simulink model "Regen1"  (Simulink 6.5)
settings: Solver=FixedStepDiscrete  StartTime=0.0  StopTime=1  FixedStep=Ts  RelTol=1e-3  AbsTol=1e-3
PreLoadFcn:
  | assignin('base','Ts',[2e-6])
undefined symbols (not defined in the file): DiscIntNeverNeededParam, powergui, Ts, x
libraries: powerlib x18, powerlib_extras x8
settings Model: Creator=sybille  LastModifiedBy=RS  ExtModeTrigMode=oneshot  ExtModeArmWhenConnect=off  ExtModeAutoUpdateStatusClock=off
settings DataIOCC: LimitDataPoints=off  SaveOutput=off  SaveTime=off  SignalLoggingName=sigsOut
settings OptimizationCC: BlockReduction=off  BooleanDataType=off  InlineInvariantSignals=on
settings DebuggingCC: CheckExecutionContextPreStartOutputMsg=on  CheckExecutionContextRuntimeOutputMsg=on  SolverPrmCheckMsg=none  MultiTaskDSMMsg=warning  MultiTaskCondExecSysMsg=none  StrictBusMsg=None
settings HardwareCC: TargetUnknown=on
settings RTWCC: IncludeERTFirstTime=on

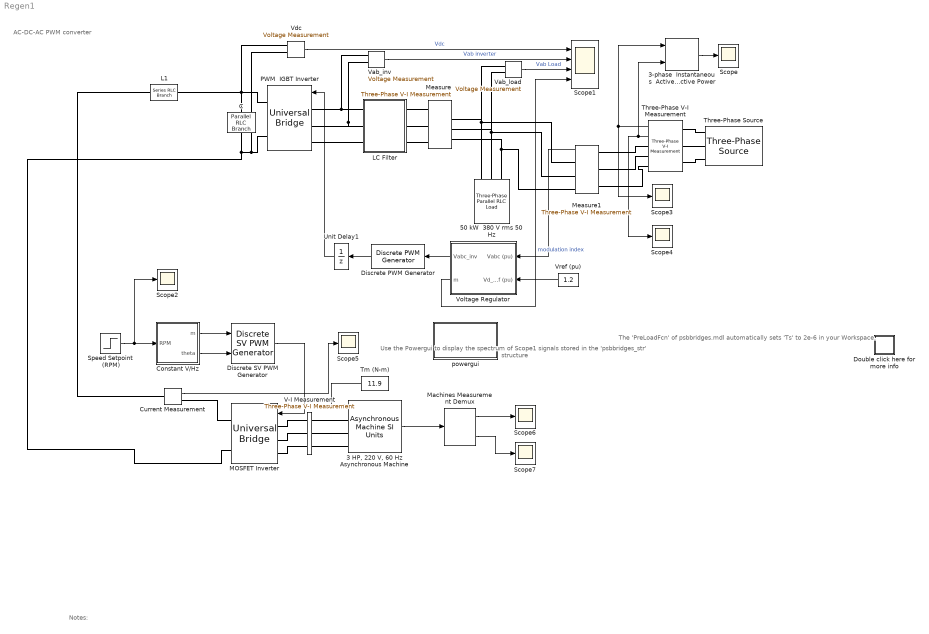
== system Regen1 ==
  note: AC-DC-AC PWM converter
  note: The 'PreLoadFcn' of psbbridges.mdl
      | automatically sets 'Ts' to 2e-6 in your Workspace.
  note: Use the Powergui to display
      | the spectrum of Scope1 signals
      | stored in the  'psbbridges_str'
      | structure
  note: Notes:
  "3 HP, 220 V, 60 Hz Asynchronous Machine" : powerlib/Machines/Asynchronous Machine SI Units  DialogController=PMDialogs.PMDefaultMaskDlg  SystemSampleTime=-1  PresetModel=No  MechanicalLoad=Torque Tm  ShowDetailedParameters=on  RotorType=Squirrel-cage  ReferenceFrame=Stationary  NominalParameters=[ 3*746, 220, 60 ]  Stator="[ 0.435  2*2.0e-3 ]"  Rotor="[ 0.816  2.0e-3 ]"  Lm=69.31e-3  Mechanical="[ 0.089  0  2 ]"  PolePairs=2  InitialConditions=[0.044533 0 11.138 11.138 11.138 -39.6 -159.6 80.4]  Units=1  LoadFlowParameters=2000  SimulateSaturation=off  Saturation=[0 0;0 0]
  3-phase  Instantaneous  Active & Reactive Power : powerlib_extras/Measurements/3-phase  Instantaneous  Active & Reactive Power  DialogController=PMDialogs.PMDefaultMaskDlg  SystemSampleTime=-1
  50 kW  380 V rms 50 Hz : powerlib/Elements/Three-Phase Parallel RLC Load  Orientation=down  DialogController=PMDialogs.PMDefaultMaskDlg  PhysicalDomain=powersysdomain  SubClassName=unknown  LeftPortType=p1  RightPortType=p1  LConnTagsString=A|B|C  Configuration=Y (grounded)  NominalVoltage=380  NominalFrequency=50  ActivePower=0  InductivePower=0  CapacitivePower=0  Measurements=None
  C : powerlib/Elements/Parallel RLC Branch  Orientation=down  DialogController=PMDialogs.PMDefaultMaskDlg  PhysicalDomain=powersysdomain  SubClassName=unknown  LeftPortType=p1  RightPortType=p1  LConnTagsString=a  RConnTagsString=__new0  BranchType=C  Resistance=1.0  Inductance=1.0  SetiL0=off  InitialCurrent=0  Capacitance=5000e-06  Setx0=off  InitialVoltage=0  Measurements=None
  Constant V/Hz : Subsystem
  Current Measurement : powerlib/Measurements/Current Measurement  DialogController=PMDialogs.PMDefaultMaskDlg  SystemSampleTime=-1  PhasorSimulation=off  OutputType=Complex  PSBequivalent=0
  Discrete PWM Generator : powerlib_extras/Discrete  Control Blocks/Discrete PWM Generator  Orientation=left  DialogController=PMDialogs.PMDefaultMaskDlg  SystemSampleTime=-1  GeneratorMode="3-arm  bridge (6 pulses)"  Fc=2000  Ts=Ts  Internal=off  mIndex=0.4  Freq=60  Phase=0
  Discrete SV PWM Generator : powerlib_extras/Discrete  Control Blocks/Discrete SV PWM Generator  DialogController=PMDialogs.PMDefaultMaskDlg  SystemSampleTime=-1  InputType=Magnitude-Angle (rad)  SwitchingPattern=Pattern #1  Fc=1980  ParUref=[0.8 -30 50]  Ts=Ts
  Double click here for more info : Subsystem
      settings: OpenFcn=showdemo(bdroot(gcb))
      mask Display: disp('?')
  L1 : powerlib/Elements/Series RLC Branch  DialogController=PMDialogs.PMDefaultMaskDlg  PhysicalDomain=powersysdomain  SubClassName=unknown  LeftPortType=p1  RightPortType=p1  LConnTagsString=__new0  RConnTagsString=__new0  BranchType=L  Resistance=1.0  Inductance=200e-6  SetiL0=off  InitialCurrent=0  Capacitance=1.0  Setx0=off  InitialVoltage=0  Measurements=None
  LC Filter : Subsystem
  MOSFET Inverter : powerlib/Power Electronics/Universal Bridge  Orientation=left  DialogController=PMDialogs.PMDefaultMaskDlg  SystemSampleTime=-1  Arms=3  SnubberResistance=1e5  SnubberCapacitance=inf  Device=MOSFET / Diodes  Ron=0.2e-3  Lon=0  ForwardVoltages="[  0  0  ]"  ForwardVoltage=0  GTOparameters=[ 10e-6 , 20e-6 ]  IGBTparameters=[ 1e-6 , 2e-6 ]  Measurements=None  converterType=Rectifier
  Machines Measurement Demux : powerlib/Machines/Machines Measurement Demux  DialogController=PMDialogs.PMDefaultMaskDlg  SystemSampleTime=-1  machType=Asynchronous  ssm1=on  ssm2=on  ssm3=on  ssm4=on  ssm5=on  ssm6=on  sm1=off  sm2=off  sm3=off  sm4=off  sm5=off  sm6=off  sm7=off  sm8=on  sm9=off  sm10=off  sm11=off  sm115=off  sm12=off  sm13=off  sm14=off  asm1=off  asm2=off  asm3=off  asm4=off  asm5=on  asm6=off  asm7=off  asm8=off  asm9=on  asm10=off  asm11=off  pmsm1=on  pmsm2=on  pmsm3=on  pmsm4=off  pmsm5=on  pmsm6=on  pmsm7=on  lastType=1
  Measure : powerlib/Measurements/Three-Phase V-I Measurement  DialogController=PMDialogs.PMDefaultMaskDlg  SystemSampleTime=-1  VoltageMeasurement=phase-to-ground  SetLabelV=off  LabelV=V1  Vpu=on  CurrentMeasurement=no  SetLabelI=off  LabelI=I1  Ipu=off  Pbase=1e3  Vbase=380  OutputType=Magnitude  PhasorSimulation=off  PSBequivalent=0
  Measure1 : powerlib/Measurements/Three-Phase V-I Measurement  Orientation=left  DialogController=PMDialogs.PMDefaultMaskDlg  SystemSampleTime=-1  VoltageMeasurement=phase-to-ground  SetLabelV=off  LabelV=V1  Vpu=on  CurrentMeasurement=no  SetLabelI=off  LabelI=I1  Ipu=off  Pbase=1e3  Vbase=380  OutputType=Magnitude  PhasorSimulation=off  PSBequivalent=0
  PWM  IGBT Inverter : powerlib/Power Electronics/Universal Bridge  Orientation=left  DialogController=PMDialogs.PMDefaultMaskDlg  SystemSampleTime=-1  Arms=3  SnubberResistance=5000  SnubberCapacitance=inf  Device=IGBT / Diodes  Ron=1e-3  Lon=0  ForwardVoltages="[  0.0  0.0  ]"  ForwardVoltage=.8  GTOparameters=[ 1e-6 ,1e-6 ]  IGBTparameters=[ 1e-6 , 2e-6 ]  Measurements=Device currents  converterType=Rectifier
  Scope{,2..7} (7 alike) : Scope
      Scope settings: MaxDataPoints=10000000  SampleInput=on  SampleTime=2e-6
      Scope2 settings: MaxDataPoints=10000000  SampleInput=on  SampleTime=2e-6
      Scope3 settings: SaveName=ScopeData2  MaxDataPoints=10000000  SampleInput=on  SampleTime=2e-6
      Scope4 settings: SaveName=ScopeData3  MaxDataPoints=10000000  SampleInput=on  SampleTime=2e-6
      Scope5 settings: SaveName=ScopeData4  MaxDataPoints=10000000  SampleInput=on  SampleTime=2e-6
      Scope6 settings: SaveName=ScopeData5  MaxDataPoints=10000000  SampleInput=on  SampleTime=2e-6
      Scope7 settings: YMin=124.5  YMax=127.25  SaveName=ScopeData6  MaxDataPoints=10000000  SampleInput=on  SampleTime=2e-6
  Scope1 : Scope  NumInputPorts=4
      settings: TimeRange=0.1  YMin=0~-1500~-750~0.4  YMax=1100~1500~750~1.1  SaveName=psbbridges_str
  Speed Setpoint (RPM) : Step  Time=0.5  After=1300  SampleTime=Ts
  Three-Phase V-I Measurement : powerlib/Measurements/Three-Phase V-I Measurement  Orientation=left  DialogController=PMDialogs.PMDefaultMaskDlg  SystemSampleTime=-1  VoltageMeasurement=phase-to-ground  SetLabelV=off  LabelV=Vabc  Vpu=off  CurrentMeasurement=yes  SetLabelI=off  LabelI=Iabc  Ipu=off  Pbase=100e6  Vbase=500e3  OutputType=Complex  PhasorSimulation=off  PSBequivalent=0
  Three-Phase Source : powerlib/Electrical Sources/Three-Phase Source  Orientation=left  DialogController=PMDialogs.PMDefaultMaskDlg  SystemSampleTime=-1  Voltage=390  PhaseAngle=0  Frequency=50  InternalConnection=Yg  SpecifyImpedance=off  Resistance=0.00001  Inductance=0.00001  ShortCircuitLevel=100e6  BaseVoltage=25e3  XRratio=7
  Tm (N-m) : Constant  Orientation=left  Value=11.9  OutDataType=sfix(16)  ConRadixGroup=Use specified scaling  OutScaling=2^0  SampleTime=inf  FramePeriod=inf
  Unit Delay1 : UnitDelay  Orientation=left  SampleTime=Ts
  V-I Measurement : powerlib/Measurements/Three-Phase V-I Measurement  DialogController=PMDialogs.PMDefaultMaskDlg  SystemSampleTime=-1  VoltageMeasurement=phase-to-phase  SetLabelV=on  LabelV=Vabc_Stator  Vpu=off  CurrentMeasurement=yes  SetLabelI=on  LabelI=Iabc_Stator  Ipu=off  Pbase=100e6  Vbase=500e3  OutputType=Magnitude  PhasorSimulation=off  PSBequivalent=0
  Vab_inv : powerlib/Measurements/Voltage Measurement  Tag=PoWeRsYsTeMmEaSuReMeNt  DialogController=PMDialogs.PMDefaultMaskDlg  SystemSampleTime=-1  PhasorSimulation=off  OutputType=Magnitude  PSBequivalent=0
  Vab_load : powerlib/Measurements/Voltage Measurement  Tag=PoWeRsYsTeMmEaSuReMeNt  DialogController=PMDialogs.PMDefaultMaskDlg  SystemSampleTime=-1  PhasorSimulation=off  OutputType=Magnitude  PSBequivalent=0
  Vdc : powerlib/Measurements/Voltage Measurement  Tag=PoWeRsYsTeMmEaSuReMeNt  DialogController=PMDialogs.PMDefaultMaskDlg  SystemSampleTime=-1  PhasorSimulation=off  OutputType=Magnitude  PSBequivalent=0
  Voltage Regulator : Subsystem  Orientation=left  mask( Voltage Regulator){Kp=0.4, Ki=500, Ts=Ts}
      mask prompts: Kp "Proportional gain  Kp:"; Ki "Integral gain Ki:"; Ts "Sample time (s) :"
  "Vref (pu) " : Constant  Orientation=left  Value=1.2  OutDataType=sfix(16)  ConRadixGroup=Use specified scaling  OutScaling=2^0  SampleTime=inf  FramePeriod=inf
  powergui : Subsystem  Priority=2  AncestorBlock=powerlib/powergui  InitFcn=powergui( 'InitFcn_Callback' , gcb , 0 , [ ] );  mask(PSB option menu block){SimulationMode=Discrete, SampleTime=Ts, echomessages=on, RestoreLinks=warning, x0status=blocks, Frange=[0:2:500], Ylog=off, Xlog=on, ShowGrid=off, save=off, variable=ZData, structure=psbbridges_str, ZoomFFT=on, StartTime=0.1-2/50, cycles=2, DisplayStyle=off, fundamental=50, FreqAxis=off, MaxFrequency=7000, frequencyindice=60, frequencyindicesteady=1, RmsSteady=1, display=off, Ts=0, frequency=60, methode=off, HookPort=off, Interpol=off}
      mask prompts: SimulationMode "Simulation mode"; SampleTime "Sample time Ts (when simulation mode is Discrete) (s)"; echomessages "Echo  Messages"; RestoreLinks "Restore disabled links"; x0status "Initial electrical states status"; Frange "Impedance tool: Frequency Range"; Ylog "Impedance tool: Log impedance"; Xlog "Impedance tool: log Frequency"; ShowGrid "Impedance tool: grid"; save "Impedance tool: Save Data To Workspace"; variable "Impedance tool: Variable Name"; structure "Structure Name (PSBFFTSCOPE)"; ZoomFFT "ZoomFFT (PSBFFTSCOPE)"; StartTime "Start Time (PSBFFTSCOPE)"; cycles "Cycles (PSBFFTSCOPE)"; DisplayStyle "Display style (PSBFFTSCOPE)"; fundamental "Fundamental (PSBFFTSCOPE)"; FreqAxis "Frequency Axis (PSBFFTSCOPE)"; MaxFrequency "Max Frequency (PSBFFTSCOPE)"; frequencyindice "Load flow frequency (Hz)"; frequencyindicesteady "Frequency indice (STEADYSTATE)"; RmsSteady "RMS display (STEADYSTATE)"; display "Display Results"; Ts "OBSOLETE 1"; frequency "Phasor frequency (Hz)"; methode "Phasor simulation"; HookPort "Hook port"; Interpol "Interpolate"
      mask init:
      | powerlibroot = which('powersysdomain');
      | PSBroot = powerlibroot(1:end-16);
      | %
      | switch SimulationMode
      | 	case 1
      | 		message=sprintf('Continuous');
      | 	case 2
      |         SampleTimeeval=evalin('base',SampleTime,'NaN');
      |         if isnan(SampleTimeeval)
      |             message=sprintf('Warning !!,\nUndefined sample time');
      |         else
      |             message=sprintf('Discrete,\nTs = %.4g s.',SampleTimeeval);
      |         end
      | 	case 3
      | 		message=sprintf('Phasors');
      | end
      | if strcmp(bdroot,'powerlib')
      |   message='powergui';
      | end
      | power_initmask();
      settings: CopyFcn=powergui( 'Copy_Callback' , gcb , 0 , [ ] );  ModelCloseFcn=powergui( 'CloseButton_Callback' , gcb , [ ] , [ ] );  PreSaveFcn=powergui( 'CloseButton_Callback' , gcb , [ ] , [ ] );  NameChangeFcn=powergui( 'NameChangeFcn_Callback' , gcb , 0 , [ ] );
      settings: DeleteFcn=|
      | powergui( 'Copy_Callback' , gcb , 1 , [ ] );
      | powergui( 'CloseButton_Callback' , gcb , [ ] , [ ] );
      settings: OpenFcn=|
      | if (power_openblockproxy ('secondary'))
      | powergui(gcb,'PM')
      | end;
      mask Help: web(psbhelp)
      mask StyleString: popup(Continuous|Discrete|Phasor),edit,checkbox,popup(yes|warning|no),popup(blocks|steady|zero),edit,checkbox,checkbox,checkbox,checkbox,edit,edit,checkbox,edit,edit,edit,edit,checkbox,edit,edit,edit,edit,checkbox,edit,edit,checkbox,checkbox,checkbox
      mask CallbackString: ||||||||||||||||||||||||||powergui('HookPort',[],[],gcb);|
      mask Display: disp(message)
  wires:
  "Vref (pu) "/1 -> Voltage Regulator/2(Vd_ref (pu))
  Discrete PWM Generator/1 -> Unit Delay1/1
  Voltage Regulator/1(Vabc_inv) -> Discrete PWM Generator/1
  Voltage Regulator/2(m) -> Scope1/4  "modulation index"
  Vdc/1 -> Scope1/1  "Vdc"
  Vab_load/1 -> Scope1/3  "Vab Load"
  Vab_inv/1 -> Scope1/2  "Vab inverter"
  Unit Delay1/1 -> PWM  IGBT Inverter/1
  3-phase  Instantaneous  Active & Reactive Power/1 -> Scope/1
  Three-Phase V-I Measurement/1 -> Scope3/1, 3-phase  Instantaneous  Active & Reactive Power/1
  Three-Phase V-I Measurement/2 -> Scope4/1, 3-phase  Instantaneous  Active & Reactive Power/2
  Measure1/1 -> Voltage Regulator/1(Vabc (pu))
  Constant V/Hz/2(theta) -> Discrete SV PWM Generator/2
  Constant V/Hz/1(m) -> Discrete SV PWM Generator/1
  Discrete SV PWM Generator/1 -> MOSFET Inverter/1
  Tm (N-m)/1 -> "3 HP, 220 V, 60 Hz Asynchronous Machine"/1
  Speed Setpoint (RPM)/1 -> Constant V/Hz/1(RPM), Scope2/1
  Current Measurement/1 -> Scope5/1
  "3 HP, 220 V, 60 Hz Asynchronous Machine"/1 -> Machines Measurement Demux/1
  Machines Measurement Demux/1 -> Scope6/1
  Machines Measurement Demux/2 -> Scope7/1
  connections:
  C/RConn1 -- PWM  IGBT Inverter/RConn2 -- Vdc/LConn2 -- MOSFET Inverter/RConn2
  C/LConn1 -- Vdc/LConn1 -- PWM  IGBT Inverter/RConn1 -- L1/RConn1
  Vab_inv/LConn2 -- PWM  IGBT Inverter/LConn2 -- LC Filter/LConn2
  Measure/RConn2 -- Vab_load/LConn2 -- 50 kW  380 V rms 50 Hz/LConn2 -- Measure1/RConn2
  Measure/RConn1 -- Vab_load/LConn1 -- 50 kW  380 V rms 50 Hz/LConn1 -- Measure1/RConn1
  50 kW  380 V rms 50 Hz/LConn3 -- Measure/RConn3 -- Measure1/RConn3
  Three-Phase Source/RConn1 -- Three-Phase V-I Measurement/LConn1
  Three-Phase Source/RConn2 -- Three-Phase V-I Measurement/LConn2
  Three-Phase Source/RConn3 -- Three-Phase V-I Measurement/LConn3
  PWM  IGBT Inverter/LConn1 -- Vab_inv/LConn1 -- LC Filter/LConn1
  LC Filter/LConn3 -- PWM  IGBT Inverter/LConn3
  LC Filter/RConn1 -- Measure/LConn1
  LC Filter/RConn2 -- Measure/LConn2
  LC Filter/RConn3 -- Measure/LConn3
  Measure1/LConn1 -- Three-Phase V-I Measurement/RConn1
  Measure1/LConn2 -- Three-Phase V-I Measurement/RConn2
  Three-Phase V-I Measurement/RConn3 -- Measure1/LConn3
  MOSFET Inverter/LConn1 -- V-I Measurement/LConn1
  Current Measurement/RConn1 -- MOSFET Inverter/RConn1
  V-I Measurement/RConn1 -- "3 HP, 220 V, 60 Hz Asynchronous Machine"/LConn1
  V-I Measurement/RConn2 -- "3 HP, 220 V, 60 Hz Asynchronous Machine"/LConn2
  V-I Measurement/RConn3 -- "3 HP, 220 V, 60 Hz Asynchronous Machine"/LConn3
  MOSFET Inverter/LConn3 -- V-I Measurement/LConn3
  MOSFET Inverter/LConn2 -- V-I Measurement/LConn2
  Current Measurement/LConn1 -- L1/LConn1

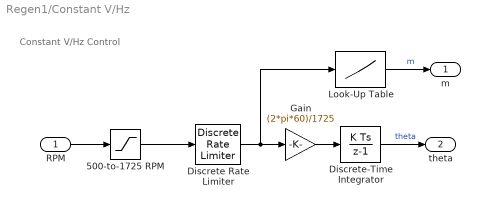
== system Regen1/Constant V/Hz ==
  note: Constant V/Hz
      | Control
  RPM : Inport
  500-to-1725 RPM : Saturate  UpperLimit=1725  LowerLimit=500
  Discrete Rate Limiter : powerlib_extras/Discrete  Control Blocks/Discrete Rate Limiter  DialogController=PMDialogs.PMDefaultMaskDlg  SystemSampleTime=-1  R=500  F=-500  Vinit=1725  Ts=Ts
  Discrete-Time Integrator : DiscreteIntegrator  SampleTime=Ts  ICPrevOutput=DiscIntNeverNeededParam  ICPrevScaledInput=DiscIntNeverNeededParam
  Gain : Gain  Gain=(2*pi*60)/1725  SaturateOnIntegerOverflow=on
  Look-Up Table : Lookup  InputValues=[500 1725 2500]  OutputValues=[0.29 1 1]*0.957  LookUpMeth=Interpolation-Extrapolation  OutDataType=sfix(16)  OutScaling=2^0  SaturateOnIntegerOverflow=on  SampleTime=-1  LUTDesignTableMode=Redesign Table  LUTDesignDataSource=Block Dialog  LUTDesignFunctionName=sqrt(x)  LUTDesignUseExistingBP=on  LUTDesignRelError=0.01  LUTDesignAbsError=1e-6  RndMeth=Floor
      settings: LockScale=off
  m : Outport
  theta : Outport  Port=2
  wires:
  Gain/1 -> Discrete-Time Integrator/1
  Discrete Rate Limiter/1 -> Gain/1, Look-Up Table/1
  Look-Up Table/1 -> m/1  "m"
  RPM/1 -> 500-to-1725 RPM/1
  Discrete-Time Integrator/1 -> theta/1  "theta"
  500-to-1725 RPM/1 -> Discrete Rate Limiter/1

== system Regen1/Double click here for more info ==
  note: This example of AC-DC-AC converter illustrates use of Universal Bridge,
      | Multimeter, and Powergui  blocks, as well as discrete control blocks of the Extras library
  note: Circuit Description
  note: Demonstration
  note: A  60 Hz, voltage source feeds a 50 Hz, 50 kW load through an  AC-DC-AC  converter.
      |
      | The 600V, 60 Hz voltage obtained at secondary of the Wye/Delta transformer is first rectified by a six pulse diode bridge.
      | The filtered DC voltage is applied to an IGBT two-level inverter generating 50 Hz.
      | The IGBT inverter uses Pulse Width Modulation (PWM) at a 2 kHz carrier frequency.
      | The circuit is discretized at a sample time of 2 us
      |
      | The load voltage is regulated at 1 pu (380 V rms) by a PI voltage regulator using abc_to_dq and dq_to_abc transfomations.
      | The first output of the voltage regulator is a vector containing the three modulating signals used by the PMW Generator
      | to generate the 6 IGBT pulses. The second output returns the modulation index.
      |
      | The Discrete 3-Phase PWM Pulse Generator is available in the Extras/Discrete Control Blocks library.
      | The voltage regulator has been  built from blocks of the Extras/Measurements and Extras/ Discrete Control libraries
      |
      | The Multimeter block is used to observe diode and IGBT currents.
      | In order to allow further signal processing, signals displayed on  Scope1 block  (sampled at simulation sampling rate of 2us )
      | are stored in a  variable named 'psbbridges_str' (structure with time) .
  note: Start the simulation. After a transient period of approximately  50 ms, the system reaches a steady state.
      | Observe  voltage waveforms at  DC bus, inverter output  and load on Scope1.
      | The harmonics generated by the inverter around around multiples of 2 kHz are filtered by the  LC filter.
      |
      | As expected the peak value of the load voltage is 537 V (380 Vrms).
      | In steady state, the mean value of the modulation index is m = 0.80 and the mean value of the  DC  voltage is 778 V.
      | The fundamental component of 50 Hz voltage burried in the chopped inverter voltage is therefore:
      | Vab = 778 V * 0.612 * 0.80 = 381 V rms
      |
      | Once  simulation is completed, open the Powergui and select  'FFT Analysis' to display the 0 - 7000 Hz frequency spectrum of signals saved
      | in the 'psbbridges_str' structure. The FFT will be performed on  a 2-cycle window starting at t=0.1-2/50 (last 2 cycles of recording).
      | Select input labeled 'Vab Load' . Click on Display and observe the frequency spectrum of last 2 cycles.
      | Notice harmonics around multiples of the 2 kHz carrier frequency. Maximum harmonic is 1.4 % of fundamental and THD is 2%.
      |
      | Observe diode currents on trace 1 of Scope2, showing commutation from  diode 1 to diode 3.  Also observe on trace 2 currents in
      | switches 1 and 2 of the IGBT/Diode bridge (upper and lower switches connected to phase A). These two currents are complementary.
      | A positive current indicates a current flowing in the IGBT, whereas a negative current indicates a current flowing in the antiparallel diode.
  note: G. Sybille (Hydro-Quebec)

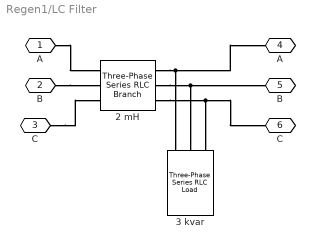
== system Regen1/LC Filter ==
  "2 mH " : powerlib/Elements/Three-Phase Series RLC Branch  DialogController=PMDialogs.PMDefaultMaskDlg  PhysicalDomain=powersysdomain  SubClassName=unknown  LeftPortType=p1  RightPortType=p1  LConnTagsString=A|B|C  RConnTagsString=A|B|C  BranchType=L  Resistance=1.0  Inductance=2e-3  Capacitance=1.0  Measurements=None
  3 kvar : powerlib/Elements/Three-Phase Series RLC Load  Orientation=down  DialogController=PMDialogs.PMDefaultMaskDlg  PhysicalDomain=powersysdomain  SubClassName=unknown  LeftPortType=p1  RightPortType=p1  LConnTagsString=A|B|C  Configuration=Y (grounded)  NominalVoltage=380  NominalFrequency=50  ActivePower=0  InductivePower=0  CapacitivePower=3e3  Measurements=None
  A : PMIOPort  Port=1  Side=Left
  B : PMIOPort  Port=2  Side=Left
  C : PMIOPort  Port=3  Side=Left
  "A " : PMIOPort  Orientation=left  Port=4  Side=Right
  "B " : PMIOPort  Orientation=left  Port=5  Side=Right
  "C " : PMIOPort  Orientation=left  Port=6  Side=Right
  connections:
  B/RConn1 -- "2 mH "/LConn2
  A/RConn1 -- "2 mH "/LConn1
  C/RConn1 -- "2 mH "/LConn3
  "2 mH "/RConn1 -- "A "/RConn1 -- 3 kvar/LConn1
  "2 mH "/RConn2 -- "B "/RConn1 -- 3 kvar/LConn2
  "2 mH "/RConn3 -- "C "/RConn1 -- 3 kvar/LConn3

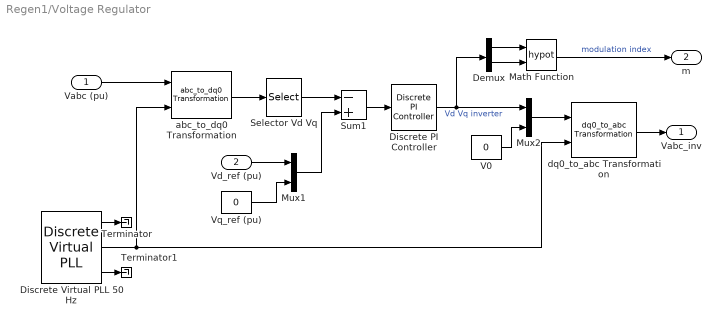
== system Regen1/Voltage Regulator ==
  Vabc (pu) : Inport
  Vd_ref (pu) : Inport  Port=2
  Demux : Demux  Outputs=2
  Discrete PI Controller : powerlib_extras/Discrete  Control Blocks/Discrete PI Controller  DialogController=PMDialogs.PMDefaultMaskDlg  SystemSampleTime=-1  Kp=Kp  Ki=Ki  Par_Limits=[1 -1]  Init=0  Ts=Ts
  Discrete Virtual PLL 50 Hz : powerlib_extras/Discrete  Control Blocks/Discrete Virtual PLL  DialogController=PMDialogs.PMDefaultMaskDlg  SystemSampleTime=-1  Freq=50  Phase=0  Ts=Ts
  Math Function : Math  Operator=hypot  SaturateOnIntegerOverflow=on
  Mux1 : Mux  Inputs=2
  Mux2 : Mux  Inputs=2
  Selector Vd Vq : Selector  InputType=Vector  ElementSrc=Internal  Elements=[1 2]  RowSrc=Internal  Rows=1  ColumnSrc=Internal  Columns=1  InputPortWidth=3  IndexIsStartValue=off
  Sum1 : Sum  Inputs=-+  SaturateOnIntegerOverflow=on  InputSameDT=on
  Terminator : Terminator
  Terminator1 : Terminator
  V0 : Constant  Value=0  OutDataType=sfix(16)  ConRadixGroup=Use specified scaling  OutScaling=2^0  SampleTime=inf  FramePeriod=inf
  Vq_ref (pu) : Constant  Value=0  OutDataType=sfix(16)  ConRadixGroup=Use specified scaling  OutScaling=2^0  SampleTime=inf  FramePeriod=inf
  abc_to_dq0 Transformation : powerlib_extras/Measurements/abc_to_dq0 Transformation  DialogController=PMDialogs.PMDefaultMaskDlg  SystemSampleTime=-1
  dq0_to_abc Transformation : powerlib_extras/Measurements/dq0_to_abc Transformation  DialogController=PMDialogs.PMDefaultMaskDlg  SystemSampleTime=-1
  Vabc_inv : Outport
  m : Outport  Port=2
  wires:
  abc_to_dq0 Transformation/1 -> Selector Vd Vq/1
  Vabc (pu)/1 -> abc_to_dq0 Transformation/1
  Selector Vd Vq/1 -> Sum1/1
  Sum1/1 -> Discrete PI Controller/1
  Mux2/1 -> dq0_to_abc Transformation/1
  V0/1 -> Mux2/2
  dq0_to_abc Transformation/1 -> Vabc_inv/1
  Discrete Virtual PLL 50 Hz/2 -> abc_to_dq0 Transformation/2, dq0_to_abc Transformation/2
  Vd_ref (pu)/1 -> Mux1/1
  Vq_ref (pu)/1 -> Mux1/2
  Mux1/1 -> Sum1/2
  Discrete Virtual PLL 50 Hz/1 -> Terminator/1
  Discrete Virtual PLL 50 Hz/3 -> Terminator1/1
  Discrete PI Controller/1 -> Demux/1, Mux2/1  "Vd Vq inverter"
  Demux/1 -> Math Function/1
  Demux/2 -> Math Function/2
  Math Function/1 -> m/1  "modulation index"

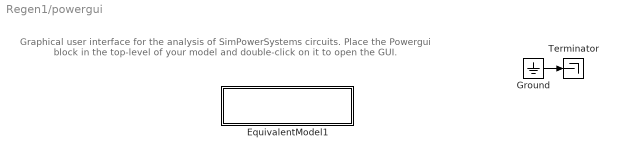
== system Regen1/powergui ==
  note: Graphical user interface for the analysis of  SimPowerSystems circuits.
      | Place the Powergui block in the top-level of your model and double-click
      | on it to open the GUI.
  EquivalentModel1 : Subsystem
      mask init:
      | SPS = get_param(gcbh,'UserData');
      | if isempty(SPS)
      | 	Ts=1;
      |     A=0;
      |     B=0;
      |     C=0;
      |     D=0;
      |     x0=0;
      |     SwitchResistance=1;
      |     SwitchType=1;
      |     SwitchGateInitialValue=1;
      |     OutputsToResetToZero=1;
      | else
      | 	Ts=SPS.PowerguiInfo.Ts;
      | 	A=SPS.Adiscrete;
      |     B=SPS.Bdiscrete;
      |     C=SPS.Cdiscrete;
      |     D=SPS.Ddiscrete;
      |     x0=SPS.x0discrete;
      |     SwitchResistance=SPS.SwitchResistance;
      |     SwitchType=SPS.SwitchType;
      |     SwitchGateInitialValue=SPS.SwitchGateInitialValue;
      |     OutputsToResetToZero=SPS.YSwitchCurrent;
      | end
      mask Display:
      | color('orange')
      | disp('EQUIVALENT CIRCUIT')
  Ground : Ground
  Terminator : Terminator
  wires:
  Ground/1 -> Terminator/1

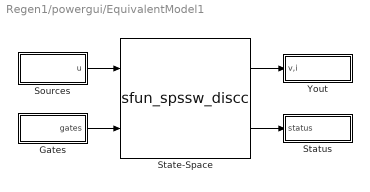
== system Regen1/powergui/EquivalentModel1 ==
  Gates : Subsystem
  Sources : Subsystem
  State-Space : S-Function  FunctionName=sfun_spssw_discc  Parameters=Ts,A, B, C, D, x0, SwitchResistance ,SwitchType, SwitchGateInitialValue, OutputsToResetToZero
  Status : Subsystem
  Yout : Subsystem
  wires:
  Gates/1(gates) -> State-Space/2
  Sources/1(u) -> State-Space/1
  State-Space/2 -> Status/1(status)
  State-Space/1 -> Yout/1(v,i)

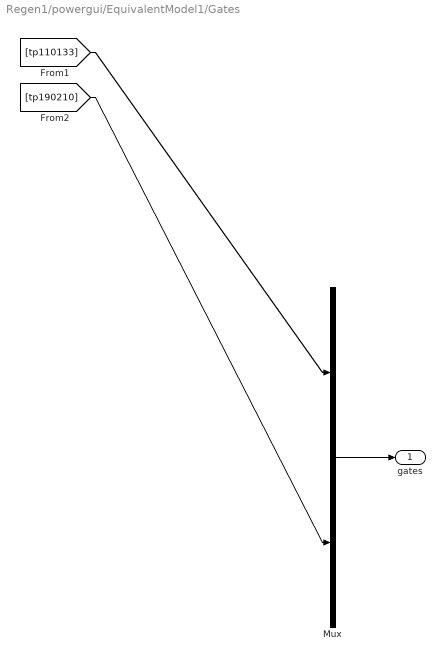
== system Regen1/powergui/EquivalentModel1/Gates ==
  Mux : Mux  Inputs=[6 6]
  gates : Outport
  wires:
  Mux/1 -> gates/1
  [tp110133] -> Mux/1
  [tp190210] -> Mux/2

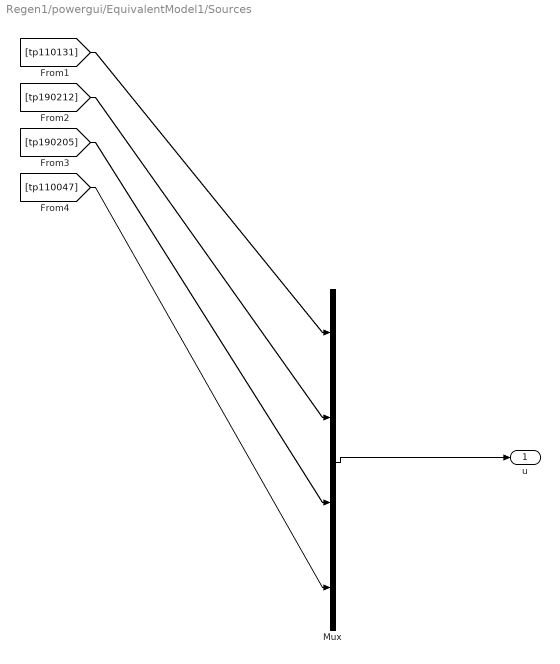
== system Regen1/powergui/EquivalentModel1/Sources ==
  Mux : Mux  Inputs=[6 6 2 3]
  u : Outport
  wires:
  Mux/1 -> u/1
  [tp110131] -> Mux/1
  [tp190212] -> Mux/2
  [tp190205] -> Mux/3
  [tp110047] -> Mux/4

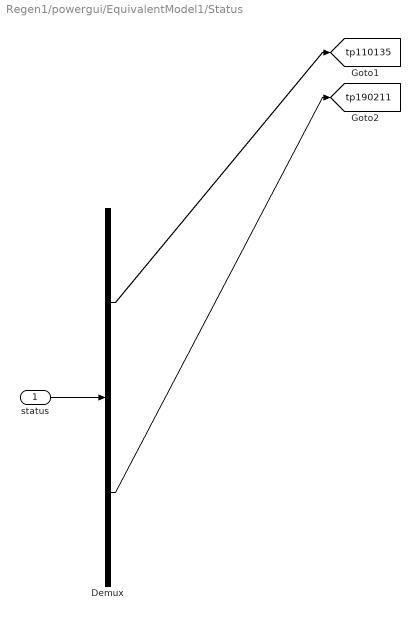
== system Regen1/powergui/EquivalentModel1/Status ==
  status : Inport
  Demux : Demux  Outputs=[6 6]
  tag scope: tp110135=global, tp190211=global
  wires:
  status/1 -> Demux/1
  Demux/1 -> [tp110135]
  Demux/2 -> [tp190211]

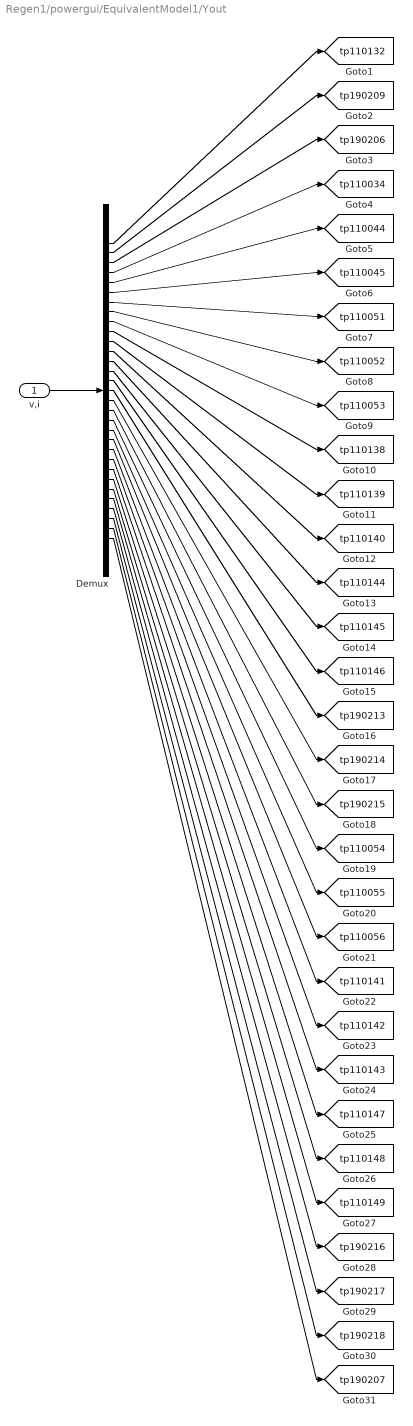
== system Regen1/powergui/EquivalentModel1/Yout ==
  v,i : Inport
  Demux : Demux  Outputs=[6 6 2 1 1 1 1 1 1 1 1 1 1 1 1 1 1 1 1 1 1 1 1 1 1 1 1 1 1 1 1]
  tag scope: tp110034=global, tp110044=global, tp110045=global, tp110051=global, tp110052=global, tp110053=global, tp110054=global, tp110055=global, tp110056=global, tp110132=global, tp110138=global, tp110139=global, tp110140=global, tp110141=global, tp110142=global, tp110143=global, tp110144=global, tp110145=global, tp110146=global, tp110147=global, tp110148=global, tp110149=global, tp190206=global, tp190207=global, tp190209=global, tp190213=global, tp190214=global, tp190215=global, tp190216=global, tp190217=global, tp190218=global
  wires:
  v,i/1 -> Demux/1
  Demux/1 -> [tp110132]
  Demux/2 -> [tp190209]
  Demux/3 -> [tp190206]
  Demux/4 -> [tp110034]
  Demux/5 -> [tp110044]
  Demux/6 -> [tp110045]
  Demux/7 -> [tp110051]
  Demux/8 -> [tp110052]
  Demux/9 -> [tp110053]
  Demux/10 -> [tp110138]
  Demux/11 -> [tp110139]
  Demux/12 -> [tp110140]
  Demux/13 -> [tp110144]
  Demux/14 -> [tp110145]
  Demux/15 -> [tp110146]
  Demux/16 -> [tp190213]
  Demux/17 -> [tp190214]
  Demux/18 -> [tp190215]
  Demux/19 -> [tp110054]
  Demux/20 -> [tp110055]
  Demux/21 -> [tp110056]
  Demux/22 -> [tp110141]
  Demux/23 -> [tp110142]
  Demux/24 -> [tp110143]
  Demux/25 -> [tp110147]
  Demux/26 -> [tp110148]
  Demux/27 -> [tp110149]
  Demux/28 -> [tp190216]
  Demux/29 -> [tp190217]
  Demux/30 -> [tp190218]
  Demux/31 -> [tp190207]
